simulink model "whs_simulin"  (R2018b)
settings: Solver=VariableStepAuto  StartTime=0.0  StopTime=39  RelTol=1e-3
settings Model: Creator=Fangming  LastModifiedBy=iamcy

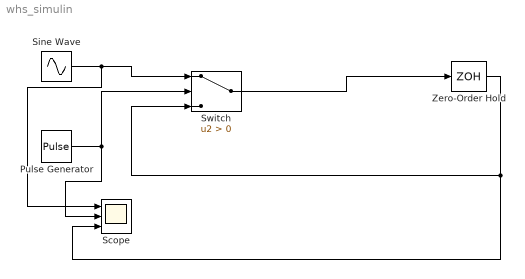
== system whs_simulin ==
  Pulse Generator : DiscretePulseGenerator  PulseType=Time based  Period=13  PulseWidth=100/13
  Scope : Scope  NumInputPorts=3
  Sine Wave : Sin  Frequency=0.01  SampleTime=0
  Switch : Switch  Criteria=u2 > Threshold
  Zero-Order Hold : ZeroOrderHold  SampleTime=13
  wires:
  Sine Wave/1 -> Scope/1, Switch/1
  Switch/1 -> Zero-Order Hold/1
  Zero-Order Hold/1 -> Scope/3, Switch/3
  Pulse Generator/1 -> Switch/2, Scope/2
